simulink model "DC_Mach2"  (Simulink 4.00)
settings: Solver=ode23tb  StartTime=0.0  StopTime=10
InitFcn:
  | powericon('psbinitsys',bdroot);
libraries: powerlib2 x3
settings Model: LastModifiedBy=ieao  BlockReductionOpt=off

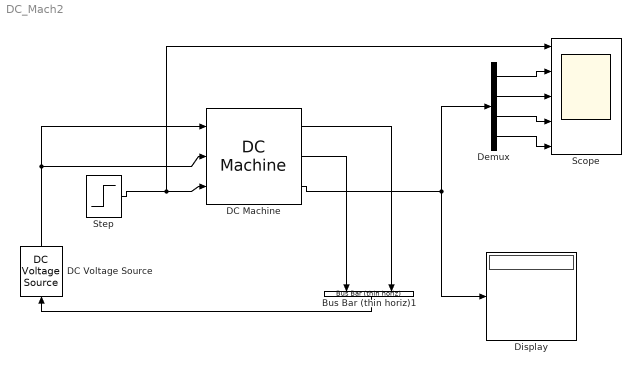
== system DC_Mach2 ==
  Bus Bar (thin horiz)1 : powerlib2/Connectors/Bus Bar (thin horiz)  Tag=PoWeRsYsTeMbLoCk  Orientation=down  input=2  output=1  PSBOutputType=111111111111111111111111111111111111111111111111111111111111111111111111111111111111
  DC Machine : powerlib2/Machines/DC Machine  RLa="[ 2.52  0.048]"  RLf=[ 92 120]  Laf=0.207  J=0.01  Bm=0  Tf=0  w0=0  PSBOutputType=110
  DC Voltage Source : powerlib2/Electrical Sources/DC Voltage Source  Tag=PoWeRsYsTeMbLoCk  Description=source block  Orientation=up  V=220  mesure=None  PSBOutputType=1
  Demux : Demux  Outputs=4  BusSelectionMode=off
  Display : Display
      settings: Format=short
  Scope : Scope  NumInputPorts=5
      settings: TimeRange=4  YMin=0~0~0~2.27174~-5  YMax=3~500~100~2.51087~5  SaveToWorkspace=off  SaveName=ScopeData  LimitDataPoints=on  MaxDataPoints=5000
  Step : Step  Time=0.01  Before=0  After=2.378  SampleTime=0
  wires:
  DC Machine/3 -> Display/1, Demux/1
  Demux/4 -> Scope/5
  Demux/3 -> Scope/4
  Demux/2 -> Scope/3
  Demux/1 -> Scope/2
  DC Voltage Source/1 -> DC Machine/2, DC Machine/1
  DC Machine/1 -> Bus Bar (thin horiz)1/2
  DC Machine/2 -> Bus Bar (thin horiz)1/1
  Bus Bar (thin horiz)1/1 -> DC Voltage Source/1
  Step/1 -> DC Machine/3, Scope/1
